simulink model "PubIfDecisionPLAN_MDL"  (R2020b)
settings: configuration reference "DspaceConfig" (kept outside this file)
PostLoadFcn:
  | if any(exist('dsrtsu_mdlpostloadfcn', 'file') ~= 0), dsrtsu_mdlpostloadfcn('Execute', bdroot); end
InitFcn:
  | , if any(exist('rtifpga_mdlclblib', 'file') ~= 0), rtifpga_mdlclblib('Init', bdroot); end,
  | , if any(exist('dsmpb_private', 'file') ~= 0), dsmpb_private('dsmpb_mdlclblib', 'Init', bdroot); end,
PreSaveFcn:
  | , if any(exist('dsmpb_private', 'file') ~= 0), dsmpb_private('dsmpb_mdlclblib', 'PreSave', bdroot); end,
CloseFcn:
  | , if any(exist('dsmpb_private', 'file') ~= 0), dsmpb_private('dsmpb_mdlclblib', 'Close', bdroot); end,
settings Model: DataDictionary=HWA_DDs.sldd  RTICANMMDATA=struct('GeneralSetupData',struct('modelroot','F:\05_dspace_Work_Files\03_HWA_Project\Git_ADAS_Store\Adas\PLAN','generalsettings',struct('filesettings',struct('destfolder',struct('Name','RTICANMM_FILES','Check',1),'buildfolder',struct('Name','.','Check',1),'AbsDestfolder',struct('Name','F:\05_dspace_Work_Files\03_HWA_Project\Git_ADAS_Store\Adas\PLAN\RTICANMM_FILES'),'AbsBuildfolder',struct('Name','F:\05_dspace_Work_Files\03_HWA_Project\Git_ADAS_Store\Adas\PLAN'))),'options',struct('addpaths',1,'rmpaths',1,'addtrcexclusion',false,'cannavigator',struct('checkmonitoring',0),'show_usrtrc',0,'use_usrtrc',0),'advanced',struct('options',ones(1,100)),'MPSetup',{{}},'RTI',struct('Type','DSRT','Ver','4.4','Date','02-Nov-2020'),'modelname','PubIfDecisionPLAN_MDL','block','PubIfDecisionPLAN_MDL'))  DSRTSU_INTERNAL_RTIFPGA=170  Creator=GW00180895  LastModifiedBy=GW00216231
settings ConfigSetRef: SourceName=DspaceConfig

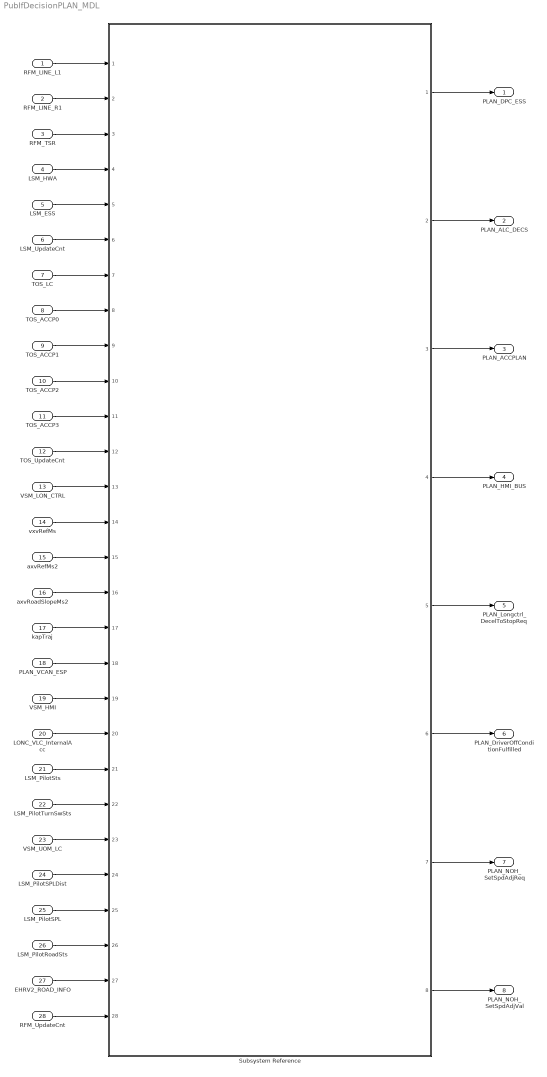
== system PubIfDecisionPLAN_MDL ==
  RFM_LINE_L1 : Inport  OutDataTypeStr=Bus: RFM_LINE_BUS  PortDimensions=1  BusOutputAsStruct=on
  RFM_LINE_R1 : Inport  Port=2  OutDataTypeStr=Bus: RFM_LINE_BUS  PortDimensions=1  BusOutputAsStruct=on
  RFM_TSR : Inport  Port=3  OutDataTypeStr=Bus: RFM_TSR_BUS  PortDimensions=1  BusOutputAsStruct=on
  LSM_HWA : Inport  Port=4  OutDataTypeStr=Bus: LSM_HWA_BUS  PortDimensions=1  BusOutputAsStruct=on
  LSM_ESS : Inport  Port=5  OutDataTypeStr=Bus: LSM_ESS_BUS  PortDimensions=1  BusOutputAsStruct=on
  LSM_UpdateCnt : Inport  Port=6  OutDataTypeStr=uint32  PortDimensions=1  BusOutputAsStruct=on
  TOS_LC : Inport  Port=7  OutDataTypeStr=Bus: TOS_LC_BUS  PortDimensions=1  BusOutputAsStruct=on
  TOS_ACCP0 : Inport  Port=8  OutDataTypeStr=Bus: TOS_ACCP0_BUS  PortDimensions=1  BusOutputAsStruct=on
  TOS_ACCP1 : Inport  Port=9  OutDataTypeStr=Bus: TOS_ACCP1_BUS  PortDimensions=1  BusOutputAsStruct=on
  TOS_ACCP2 : Inport  Port=10  OutDataTypeStr=Bus: TOS_ACCP2_BUS  PortDimensions=1  BusOutputAsStruct=on
  TOS_ACCP3 : Inport  Port=11  OutDataTypeStr=Bus: TOS_ACCP3_BUS  PortDimensions=1  BusOutputAsStruct=on
  TOS_UpdateCnt : Inport  Port=12  OutDataTypeStr=uint32  PortDimensions=1  BusOutputAsStruct=on
  VSM_LON_CTRL : Inport  Port=13  OutDataTypeStr=Bus: VSM_LON_CTRL_BUS  PortDimensions=1  BusOutputAsStruct=on
  vxvRefMs : Inport  Port=14  OutDataTypeStr=single  PortDimensions=1  BusOutputAsStruct=on
  axvRefMs2 : Inport  Port=15  OutDataTypeStr=single  PortDimensions=1  BusOutputAsStruct=on
  axvRoadSlopeMs2 : Inport  Port=16  OutDataTypeStr=single  PortDimensions=1  BusOutputAsStruct=on
  kapTraj : Inport  Port=17  OutDataTypeStr=single  PortDimensions=1  BusOutputAsStruct=on
  PLAN_VCAN_ESP : Inport  Port=18  OutDataTypeStr=Bus: VCAN_ESP_MSG_BUS  PortDimensions=1  BusOutputAsStruct=on
  VSM_HMI : Inport  Port=19  OutDataTypeStr=Bus: VSM_HMI_BUS  PortDimensions=1  BusOutputAsStruct=on
  LONC_VLC_InternalAcc : Inport  Port=20  OutDataTypeStr=single  PortDimensions=1  BusOutputAsStruct=on
  LSM_PilotSts : Inport  Port=21  OutDataTypeStr=uint8  PortDimensions=1  BusOutputAsStruct=on
  LSM_PilotTurnSwSts : Inport  Port=22  OutDataTypeStr=uint8  PortDimensions=1  BusOutputAsStruct=on
  VSM_UOM_LC : Inport  Port=23  OutDataTypeStr=Bus: VSM_UOM_LC_BUS  PortDimensions=1  BusOutputAsStruct=on
  LSM_PilotSPLDist : Inport  Port=24  OutDataTypeStr=uint16
  LSM_PilotSPL : Inport  Port=25  OutDataTypeStr=uint8
  LSM_PilotRoadSts : Inport  Port=26  OutDataTypeStr=uint8
  EHRV2_ROAD_INFO : Inport  Port=27  OutDataTypeStr=Bus: EHRV2_ROAD_INFO_BUS
  RFM_UpdateCnt : Inport  Port=28
  Subsystem Reference : Subsystem  ReferencedSubsystem=PvtSubSys_PLAN_ALL
  PLAN_DPC_ESS : Outport  OutDataTypeStr=Bus: PLAN_DPC_ESS_BUS  PortDimensions=1  BusOutputAsStruct=on
  PLAN_ALC_DECS : Outport  Port=2  OutDataTypeStr=Bus: PLAN_ALC_DECS_BUS  PortDimensions=1  BusOutputAsStruct=on
  PLAN_ACCPLAN : Outport  Port=3  OutDataTypeStr=Bus: PLAN_ACCPLAN_BUS  PortDimensions=1  BusOutputAsStruct=on
  PLAN_HMI_BUS : Outport  Port=4  OutDataTypeStr=Bus: PLAN_HMI_BUS
  PLAN_Longctrl_DecelToStopReq : Outport  Port=5  OutDataTypeStr=boolean
  PLAN_DriverOffConditionFulfilled : Outport  Port=6  OutDataTypeStr=boolean
  PLAN_NOH_SetSpdAdjReq : Outport  Port=7  OutDataTypeStr=boolean
  PLAN_NOH_SetSpdAdjVal : Outport  Port=8  OutDataTypeStr=uint8
  wires:
  RFM_LINE_L1/1 -> Subsystem Reference/1
  RFM_LINE_R1/1 -> Subsystem Reference/2
  RFM_TSR/1 -> Subsystem Reference/3
  LSM_HWA/1 -> Subsystem Reference/4
  LSM_ESS/1 -> Subsystem Reference/5
  LSM_UpdateCnt/1 -> Subsystem Reference/6
  TOS_LC/1 -> Subsystem Reference/7
  TOS_ACCP0/1 -> Subsystem Reference/8
  TOS_ACCP1/1 -> Subsystem Reference/9
  TOS_ACCP2/1 -> Subsystem Reference/10
  TOS_ACCP3/1 -> Subsystem Reference/11
  TOS_UpdateCnt/1 -> Subsystem Reference/12
  VSM_LON_CTRL/1 -> Subsystem Reference/13
  vxvRefMs/1 -> Subsystem Reference/14
  axvRefMs2/1 -> Subsystem Reference/15
  axvRoadSlopeMs2/1 -> Subsystem Reference/16
  kapTraj/1 -> Subsystem Reference/17
  PLAN_VCAN_ESP/1 -> Subsystem Reference/18
  VSM_HMI/1 -> Subsystem Reference/19
  LSM_PilotSts/1 -> Subsystem Reference/21
  LSM_PilotTurnSwSts/1 -> Subsystem Reference/22
  VSM_UOM_LC/1 -> Subsystem Reference/23
  Subsystem Reference/1 -> PLAN_DPC_ESS/1
  Subsystem Reference/3 -> PLAN_ACCPLAN/1
  Subsystem Reference/2 -> PLAN_ALC_DECS/1
  LONC_VLC_InternalAcc/1 -> Subsystem Reference/20
  Subsystem Reference/4 -> PLAN_HMI_BUS/1
  Subsystem Reference/5 -> PLAN_Longctrl_DecelToStopReq/1
  Subsystem Reference/6 -> PLAN_DriverOffConditionFulfilled/1
  LSM_PilotSPLDist/1 -> Subsystem Reference/24
  LSM_PilotSPL/1 -> Subsystem Reference/25
  LSM_PilotRoadSts/1 -> Subsystem Reference/26
  Subsystem Reference/7 -> PLAN_NOH_SetSpdAdjReq/1
  Subsystem Reference/8 -> PLAN_NOH_SetSpdAdjVal/1
  EHRV2_ROAD_INFO/1 -> Subsystem Reference/27
  RFM_UpdateCnt/1 -> Subsystem Reference/28
